simulink model "rtwdemo_deadpath"  (Simulink 7.6)
settings: Solver=FixedStepDiscrete  StartTime=0.0  StopTime=10.0  FixedStep=1  RelTol=1e-3
libraries: rtwdemowidgets x2
Description:
  | Dead Path Elimination
settings Model: Creator=The MathWorks Inc.  ExtModeAutoUpdateStatusClock=off
settings MATStruct: SampleTime=1  Offset=0  Priority=[20.0]
settings DataIOCC: SaveOutput=off  SaveTime=off  SignalLoggingName=sigsOut
settings OptimizationCC: InlineParams=on  InlineInvariantSignals=on  StateBitsets=on  DataBitsets=on  UseTempVars=on  EfficientFloat2IntCast=on  EfficientMapNaN2IntZero=off
settings DebuggingCC: CheckExecutionContextPreStartOutputMsg=on  CheckExecutionContextRuntimeOutputMsg=on  SolverPrmCheckMsg=none  StrictBusMsg=ErrorOnBusTreatedAsVector
settings HardwareCC: ProdIntDivRoundTo=Zero  ProdEndianess=LittleEndian  ProdHWDeviceType=Generic->32-bit Embedded Processor  TargetHWDeviceType=Generic->32-bit Embedded Processor
settings RTWCC: TLCOptions=-p0 -aWarnNonSaturatedBlocks=0  GenerateReport=on  RTWVerbose=off  ProcessScript=grt_make_rtw_hook  LaunchReport=on
settings CodeAppCC: ForceParamTrailComments=on
settings GRTTargetCC: TargetFcnLib=ansi_tfl_tmw.mat

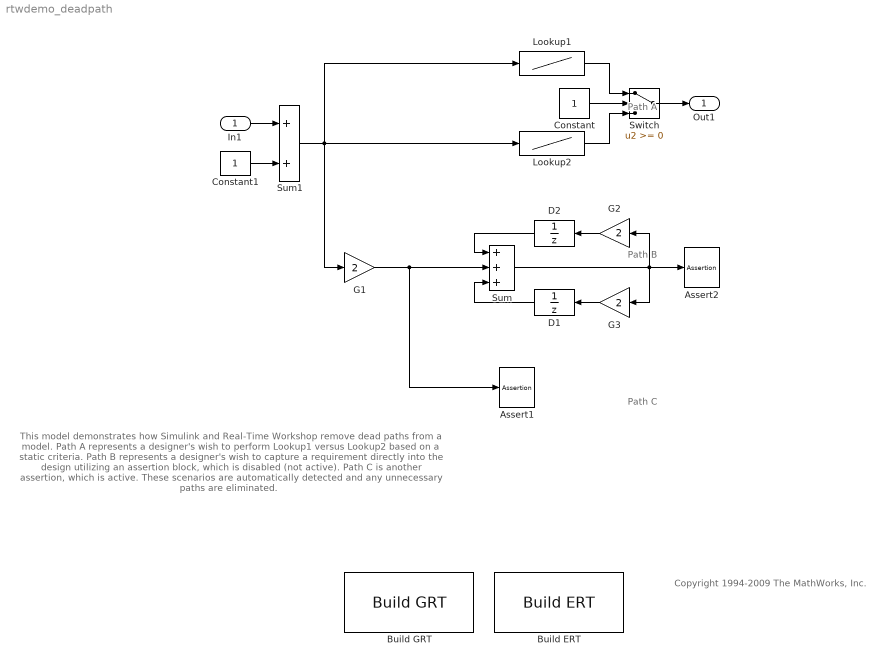
== system rtwdemo_deadpath ==
  note: This model demonstrates how Simulink and Real-Time Workshop remove dead paths from a model.
      | Path A represents a designer's wish to perform Lookup1 versus Lookup2 based on a static criteria.
      | Path B represents a designer's wish to capture a requirement directly into the design utilizing an
      | assertion block, which is disabled (not active).  Path C is another  assertion, which is active.
      | These scenarios are automatically detected and any unnecessary paths are eliminated.
  note: Path B
  note: Path C
  note: Path A
  note: Copyright 1994-2009 The MathWorks, Inc.
  In1 : Inport  OutDataTypeStr=double  PortDimensions=1  SampleTime=1
  Assert1 : Assertion  Enabled=on
  Assert2 : Assertion  Enabled=off
  Build ERT : rtwdemowidgets/Build ERT  SystemSampleTime=-1  attrib_overrides={}
  Build GRT : rtwdemowidgets/Build GRT  SystemSampleTime=-1  attrib_overrides={}
  Constant : Constant
  Constant1 : Constant
  D1 : UnitDelay
  D2 : UnitDelay
  G1 : Gain  Gain=2  SaturateOnIntegerOverflow=on  OutDataTypeStr=Inherit: Same as input  ParamDataTypeStr=Inherit: Same as input
  G2 : Gain  Gain=2  SaturateOnIntegerOverflow=on  OutDataTypeStr=Inherit: Same as input  ParamDataTypeStr=Inherit: Same as input
  G3 : Gain  Gain=2  SaturateOnIntegerOverflow=on  OutDataTypeStr=Inherit: Same as input  ParamDataTypeStr=Inherit: Same as input
  Lookup1 : Lookup  InputValues=[-5:5]  Table=tanh([-5:5])  SaturateOnIntegerOverflow=on
  Lookup2 : Lookup  InputValues=[-5:5]  Table=cosh([-5:5])  SaturateOnIntegerOverflow=on
  Sum : Sum  Inputs=+++  SaturateOnIntegerOverflow=on
  Sum1 : Sum  SaturateOnIntegerOverflow=on
  Switch : Switch  SaturateOnIntegerOverflow=on
  Out1 : Outport
  wires:
  Constant/1 -> Switch/2
  Lookup1/1 -> Switch/1
  Lookup2/1 -> Switch/3
  Switch/1 -> Out1/1
  Sum1/1 -> Lookup1/1, Lookup2/1, G1/1
  G1/1 -> Sum/2, Assert1/1
  D2/1 -> Sum/1
  G2/1 -> D2/1
  D1/1 -> Sum/3
  G3/1 -> D1/1
  Sum/1 -> G3/1, G2/1, Assert2/1
  In1/1 -> Sum1/1
  Constant1/1 -> Sum1/2
